simulink model "ss1_inter"  (R2019a)
settings: Solver=ode14x  StartTime=beginTime  StopTime=0.456  FixedStep=1e-4  RelTol=1e-3  EnableMultiTasking=on
model workspace (MAT data in the model file):
  Ankle_L_D = 1.86999822456
  Ankle_L_S = 0.0237763920936
  Ankle_R_D = 0.0588397140494
  Ankle_R_S = 0.739584271752
  F_C = 0.0618
  F_H = 0.107
  F_I = 0.0129
  F_L = 0.2471
  F_M = 1.2499
  F_W = 0.11
  GRF_HD = 42097.5090581
  GRF_HS = 111995.804745
  GRF_VD = 23523.4518935
  GRF_VS = 88551.3661398
  HAT_I = 4.3688
  HAT_L = 0.549
  HAT_M = 58.9182
  HAT_a = 0.2
  HAT_b = 0.13
  Hip_L_D = 0.00120944164738
  Hip_L_S = 1.91959156409
  Hip_R_D = 0.00174333284727
  Hip_R_S = 0.483982271561
  Knee_L_D = 0.900041230997
  Knee_L_S = 0.0187606009115
  Knee_R_D = 0.0722123401531
  Knee_R_S = 0.0187606009115
  M : struct (value not decoded)
  S_I = 0.073
  S_L = 0.447
  S_M = 4.0083
  S_R1 = 0.06
  S_R2 = 0.08
  T_I = 0.2042
  T_L = 0.476
  T_M = 8.62
  T_R1 = 0.08
  T_R2 = 0.1
  beginTime = 0.0166
  bodymass = 86.2
  lagStanceAnkle = [0 0 0 0 0 0]
  lagSwingAnkle = [0 0 0 0 0 0]
  lagSwingHip = [0 0 0 0 0 0]
  lagSwingKnee = [0 0 0 0 0 0]
  p_stance_ankle_i = 3.55817508048
  p_stance_hip_i = 23.7121133444
  p_stance_knee_i = -14.6552485707
  p_swing_ankle_i = -35.5709727014
  p_swing_hip_i = -19.0699177299
  p_swing_knee_i = -0.711619105868
  polyfit_stance_ankle = [23675.5212354 -31931.2429023 15252.5151968 -3621.5696911 268.973048302 -0.00762323811385]
  polyfit_swing_ankle = [-7183170.28304 10168157.4246 -5826762.40795 1748786.50975 -298844.069674 29567.8455925 -1567.7731554 24.418061318 1.56689555274]
  polyfit_swing_hip = [-184063768.654 261180473.575 -149801561.895 44513131.158 -7279965.6736 635960.536344 -25237.4588361 73.5247488612 22.0195049052]
  polyfit_swing_knee = [-121821446.299 173842986.405 -100273096.775 30000313.7158 -4970023.76394 451012.243214 -20836.4993451 353.694972881 6.37011560058]
  w_stance_ankle_i = 20.2190235478
  w_stance_hip_i = -62.2867196647
  w_stance_knee_i = -17.283984408
  w_swing_ankle_i = -338.75780931
  w_swing_hip_i = -1.73082510839
  w_swing_knee_i = 5.84839810815
  x_planar_p_i = -1.2363122322e-07
  x_planar_v_i = -5.51222083642e-05
  y_planar_p_i = -5.63070475942e-05
  y_planar_v_i = -0.0311861663822
  z_planar_p_i = 0.00649080902233
  z_planar_v_i = 3.33643661494
symbols that are objects in the model workspace (value not decoded): M
undefined symbols (not defined in the file or in its folder): X, Y, Z
libraries: nesl_utility x60, sm_lib x46, fl_lib x24, fl_ps_legacy_lib x14
(part 5 of 7)

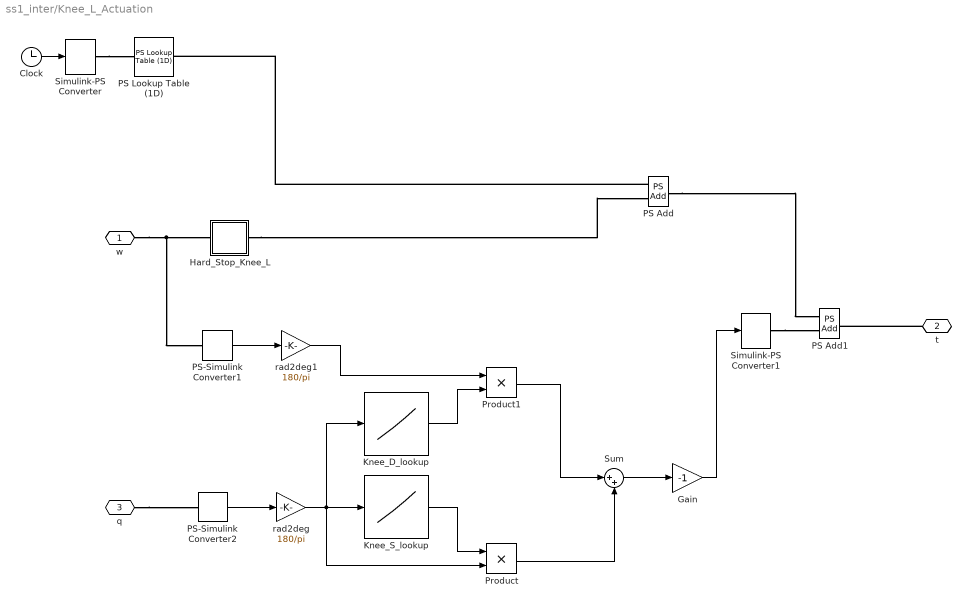
== system ss1_inter/Knee_L_Actuation ==
  Clock : Clock
  Gain : Gain  Gain=-1
  Hard_Stop_Knee_L : Subsystem  mask{upper_bound=(-p_stance_knee_i*pi)/180, lower_bound=((-140-p_stance_knee_i)*pi)/180, contact_stiffness=1e8, contact_damping=5000, initial_angular_position=0}
      mask prompts: upper_bound "Upper Bound"; lower_bound "Lower Bound"; contact_stiffness "Contact Stiffness"; contact_damping "Contact Damping"; initial_angular_position "Initial Angular Position"
  Knee_D_lookup : Lookup_n-D  NumberOfTableDimensions=1  BreakpointsForDimension1=[-140:.01:0]  Table=[exp(linspace(log(1000),log(.01),1000)), zeros(1,12000),exp(linspace(log(.01),log(1000),1001))]  RndMeth=Simplest  InputSameDT=on
  Knee_S_lookup : Lookup_n-D  NumberOfTableDimensions=1  BreakpointsForDimension1=[-140:.01:0]  Table=[exp(linspace(log(10000),log(.01),1000)), zeros(1,12000),exp(linspace(log(.01),log(10000),1001))]  RndMeth=Simplest  InputSameDT=on
  PS Add : fl_ps_legacy_lib/Legacy Physical Signals/Functions/PS Add
      settings: SourceProductName=Simscape  SourceProductBaseCode=SS
  PS Add1 : fl_ps_legacy_lib/Legacy Physical Signals/Functions/PS Add
      settings: SourceProductName=Simscape  SourceProductBaseCode=SS
  PS Lookup Table (1D) : fl_ps_legacy_lib/Legacy Physical Signals/Lookup Tables/PS Lookup Table (1D)  x=linspace(0,.3917,47)'  f=(-M.stance_knee_av/1000)*bodymass  interp_method=2  extrap_method=1
      settings: SourceProductName=Simscape  SourceProductBaseCode=SS
  PS-Simulink Converter1 : nesl_utility/PS-Simulink Converter  PhysicalDomain=network_engine_domain  SubClassName=ps_output  LeftPortType=input  RightPortType=output  PseudoPeriodic=off  Frequencies=[]  Unit=1  AffineConversion=off
  PS-Simulink Converter2 : nesl_utility/PS-Simulink Converter  PhysicalDomain=network_engine_domain  SubClassName=ps_output  LeftPortType=input  RightPortType=output  PseudoPeriodic=off  Frequencies=[]  Unit=1  AffineConversion=off
  Product : Product  RndMeth=Zero
  Product1 : Product  RndMeth=Zero
  Simulink-PS Converter : nesl_utility/Simulink-PS Converter  PhysicalDomain=network_engine_domain  SubClassName=ps_input  LeftPortType=input  RightPortType=output  PseudoPeriodic=off  Frequencies=[]  NoiseDistribution=none  NoiseParameters=[]  Unit=1  AffineConversion=off  FilteringAndDerivatives=zero  SimscapeFilterOrder=1  InputFilterTimeConstant=.001  UdotUserProvided=[]
  Simulink-PS Converter1 : nesl_utility/Simulink-PS Converter  PhysicalDomain=network_engine_domain  SubClassName=ps_input  LeftPortType=input  RightPortType=output  PseudoPeriodic=off  Frequencies=[]  NoiseDistribution=none  NoiseParameters=[]  Unit=1  AffineConversion=off  FilteringAndDerivatives=zero  SimscapeFilterOrder=1  InputFilterTimeConstant=.001  UdotUserProvided=[]
  Sum : Sum  Inputs=|++
  rad2deg : Gain  Gain=180/pi
  "rad2deg1 " : Gain  Gain=180/pi
  w : PMIOPort  Side=Right
  t : PMIOPort  Port=2  Side=Left
  q : PMIOPort  Port=3  Side=Right
  wires:
  Clock/1 -> Simulink-PS Converter/1
  PS-Simulink Converter1/1 -> "rad2deg1 "/1
  PS-Simulink Converter2/1 -> rad2deg/1
  rad2deg/1 -> Knee_S_lookup/1, Knee_D_lookup/1, Product/2
  Knee_S_lookup/1 -> Product/1
  "rad2deg1 "/1 -> Product1/1
  Product1/1 -> Sum/1
  Product/1 -> Sum/2
  Sum/1 -> Gain/1
  Gain/1 -> Simulink-PS Converter1/1
  Knee_D_lookup/1 -> Product1/2
  connections:
  Hard_Stop_Knee_L/RConn1 -- PS Add/LConn2
  w/RConn1 -- PS-Simulink Converter1/LConn1 -- Hard_Stop_Knee_L/LConn1
  Simulink-PS Converter/RConn1 -- PS Lookup Table (1D)/LConn1
  t/RConn1 -- PS Add1/RConn1
  q/RConn1 -- PS-Simulink Converter2/LConn1
  PS Add/RConn1 -- PS Add1/LConn1
  Simulink-PS Converter1/RConn1 -- PS Add1/LConn2
  PS Add/LConn1 -- PS Lookup Table (1D)/RConn1

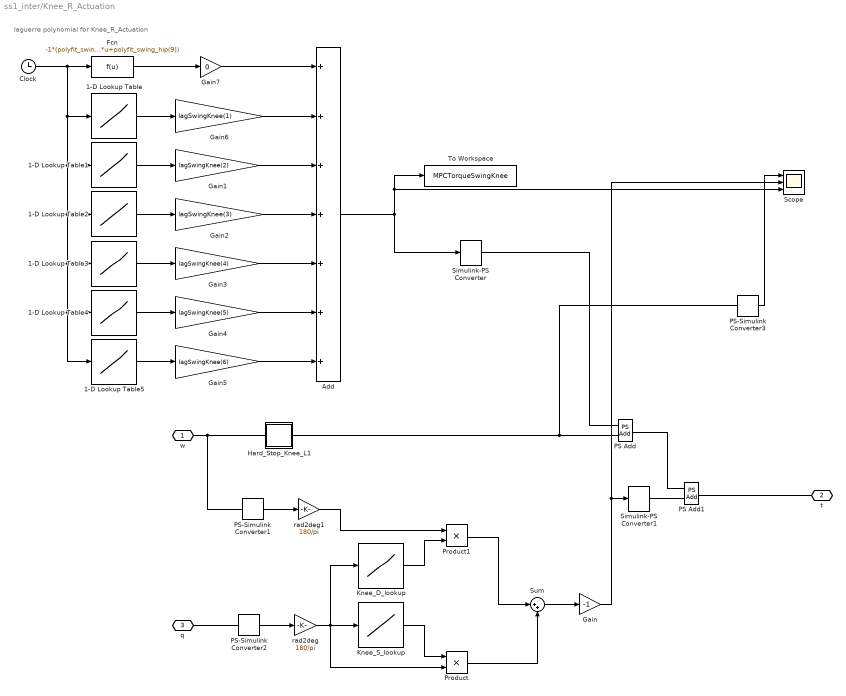
== system ss1_inter/Knee_R_Actuation ==
  note: laguerre polynomial for Knee_R_Actuation
  1-D Lookup Table : Lookup_n-D  NumberOfTableDimensions=1  BreakpointsForDimension1=|  Table=|  InternalRulePriority=Speed  RndMeth=Simplest  InputSameDT=on
      BreakpointsForDimension1=|
      | [0
      | 0.00500000000000000
      | 0.0100000000000000
      | 0.0150000000000000
      | 0.0200000000000000
      | 0.0250000000000000
      | 0.0300000000000000
      | 0.0350000000000000
      | 0.0400000000000000
      | 0.0450000000000000
      | 0.0500000000000000
      | 0.0550000000000000
      | 0.0600000000000000
      | 0.0650000000000000
      | 0.0700000000000000
      | 0.0750000000000000
      | 0.0800000000000000
      | 0.0850000000000000
      | 0.0900000000000000
      | 0.0950000000000000
      | 0.100000000000000
      | 0.105000000000000
      | 0.110000000000000
      | 0.115000000000000
      | 0.120000000000000
      | 0.125000000000000
      | 0.130000000000000
      | 0.135000000000000
      | 0.140000000000000
      | 0.145000000000000
      | 0.150000000000000
      | 0.155000000000000
      | 0.160000000000000
      | 0.165000000000000
      | 0.170000000000000
      | 0.175000000000000
      | 0.180000000000000
      | 0.185000000000000
      | 0.190000000000000
      | 0.195000000000000
      | 0.200000000000000
      | 0.205000000000000
      | 0.210000000000000
      | 0.215000000000000
      | 0.220000000000000
      | 0.225000000000000
      | 0.230000000000000
      | 0.235000000000000
      | 0.240000000000000
      | 0.245000000000000
      | 0.250000000000000
      | 0.255000000000000
      | 0.260000000000000
      | 0.265000000000000
      | 0.270000000000000
      | 0.275000000000000
      | 0.280000000000000
      | 0.285000000000000
      | 0.290000000000000
      | 0.295000000000000
      | 0.300000000000000
      | 0.305000000000000
      | 0.310000000000000
      | 0.315000000000000
      | 0.320000000000000
      | 0.325000000000000
      | 0.330000000000000
      | 0.335000000000000
      | 0.340000000000000
      | 0.345000000000000
      | 0.350000000000000
      | 0.355000000000000
      | 0.360000000000000
      | 0.365000000000000
      | 0.370000000000000
      | 0.375000000000000
      | 0.380000000000000
      | 0.385000000000000
      | 0.390000000000000
      | 0.395000000000000
      | 0.400000000000000
      | 0.405000000000000
      | 0.410000000000000
      | 0.415000000000000
      | 0.420000000000000
      | 0.425000000000000
      | 0.430000000000000
      | 0.435000000000000
      | 0.440000000000000
      | 0.445000000000000
      | 0.450000000000000
      | 0.455000000000000
      | 0.460000000000000
      | 0.465000000000000
      | 0.470000000000000
      | 0.475000000000000
      | 0.480000000000000
      | 0.485000000000000
      | 0.490000000000000
      | 0.495000000000000
      | 0.500000000000000]
      Table=|
      | [1
      | 0.800000000000000
      | 0.640000000000000
      | 0.512000000000000
      | 0.409600000000000
      | 0.327680000000000
      | 0.262144000000000
      | 0.209715200000000
      | 0.167772160000000
      | 0.134217728000000
      | 0.107374182400000
      | 0.0858993459200001
      | 0.0687194767360000
      | 0.0549755813888000
      | 0.0439804651110400
      | 0.0351843720888320
      | 0.0281474976710656
      | 0.0225179981368525
      | 0.0180143985094820
      | 0.0144115188075856
      | 0.0115292150460685
      | 0.00922337203685479
      | 0.00737869762948383
      | 0.00590295810358706
      | 0.00472236648286965
      | 0.00377789318629572
      | 0.00302231454903658
      | 0.00241785163922926
      | 0.00193428131138341
      | 0.00154742504910673
      | 0.00123794003928538
      | 0.000990352031428306
      | 0.000792281625142645
      | 0.000633825300114116
      | 0.000507060240091293
      | 0.000405648192073034
      | 0.000324518553658427
      | 0.000259614842926742
      | 0.000207691874341394
      | 0.000166153499473115
      | 0.000132922799578492
      | 0.000106338239662794
      | 8.50705917302348e-05
      | 6.80564733841879e-05
      | 5.44451787073503e-05
      | 4.35561429658802e-05
      | 3.48449143727042e-05
      | 2.78759314981633e-05
      | 2.23007451985307e-05
      | 1.78405961588245e-05
      | 1.42724769270596e-05
      | 1.14179815416477e-05
      | 9.13438523331817e-06
      | 7.30750818665453e-06
      | 5.84600654932363e-06
      | 4.67680523945890e-06
      | 3.74144419156712e-06
      | 2.99315535325370e-06
      | 2.39452428260296e-06
      | 1.91561942608237e-06
      | 1.53249554086589e-06
      | 1.22599643269272e-06
      | 9.80797146154172e-07
      | 7.84637716923338e-07
      | 6.27710173538670e-07
      | 5.02168138830936e-07
      | 4.01734511064749e-07
      | 3.21387608851799e-07
      | 2.57110087081439e-07
      | 2.05688069665152e-07
      | 1.64550455732121e-07
      | 1.31640364585697e-07
      | 1.05312291668558e-07
      | 8.42498333348461e-08
      | 6.73998666678769e-08
      | 5.39198933343015e-08
      | 4.31359146674412e-08
      | 3.45087317339530e-08
      | 2.76069853871624e-08
      | 2.20855883097299e-08
      | 1.76684706477839e-08
      | 1.41347765182271e-08
      | 1.13078212145817e-08
      | 9.04625697166537e-09
      | 7.23700557733230e-09
      | 5.78960446186584e-09
      | 4.63168356949267e-09
      | 3.70534685559414e-09
      | 2.96427748447531e-09
      | 2.37142198758025e-09
      | 1.89713759006420e-09
      | 1.51771007205136e-09
      | 1.21416805764109e-09
      | 9.71334446112870e-10
      | 7.77067556890296e-10
      | 6.21654045512237e-10
      | 4.97323236409790e-10
      | 3.97858589127832e-10
      | 3.18286871302265e-10
      | 2.54629497041812e-10
      | 2.03703597633450e-10]
  1-D Lookup Table1 : Lookup_n-D  NumberOfTableDimensions=1  BreakpointsForDimension1=|  Table=|  InternalRulePriority=Speed  RndMeth=Simplest  InputSameDT=on
      BreakpointsForDimension1=|
      | [0
      | 0.00500000000000000
      | 0.0100000000000000
      | 0.0150000000000000
      | 0.0200000000000000
      | 0.0250000000000000
      | 0.0300000000000000
      | 0.0350000000000000
      | 0.0400000000000000
      | 0.0450000000000000
      | 0.0500000000000000
      | 0.0550000000000000
      | 0.0600000000000000
      | 0.0650000000000000
      | 0.0700000000000000
      | 0.0750000000000000
      | 0.0800000000000000
      | 0.0850000000000000
      | 0.0900000000000000
      | 0.0950000000000000
      | 0.100000000000000
      | 0.105000000000000
      | 0.110000000000000
      | 0.115000000000000
      | 0.120000000000000
      | 0.125000000000000
      | 0.130000000000000
      | 0.135000000000000
      | 0.140000000000000
      | 0.145000000000000
      | 0.150000000000000
      | 0.155000000000000
      | 0.160000000000000
      | 0.165000000000000
      | 0.170000000000000
      | 0.175000000000000
      | 0.180000000000000
      | 0.185000000000000
      | 0.190000000000000
      | 0.195000000000000
      | 0.200000000000000
      | 0.205000000000000
      | 0.210000000000000
      | 0.215000000000000
      | 0.220000000000000
      | 0.225000000000000
      | 0.230000000000000
      | 0.235000000000000
      | 0.240000000000000
      | 0.245000000000000
      | 0.250000000000000
      | 0.255000000000000
      | 0.260000000000000
      | 0.265000000000000
      | 0.270000000000000
      | 0.275000000000000
      | 0.280000000000000
      | 0.285000000000000
      | 0.290000000000000
      | 0.295000000000000
      | 0.300000000000000
      | 0.305000000000000
      | 0.310000000000000
      | 0.315000000000000
      | 0.320000000000000
      | 0.325000000000000
      | 0.330000000000000
      | 0.335000000000000
      | 0.340000000000000
      | 0.345000000000000
      | 0.350000000000000
      | 0.355000000000000
      | 0.360000000000000
      | 0.365000000000000
      | 0.370000000000000
      | 0.375000000000000
      | 0.380000000000000
      | 0.385000000000000
      | 0.390000000000000
      | 0.395000000000000
      | 0.400000000000000
      | 0.405000000000000
      | 0.410000000000000
      | 0.415000000000000
      | 0.420000000000000
      | 0.425000000000000
      | 0.430000000000000
      | 0.435000000000000
      | 0.440000000000000
      | 0.445000000000000
      | 0.450000000000000
      | 0.455000000000000
      | 0.460000000000000
      | 0.465000000000000
      | 0.470000000000000
      | 0.475000000000000
      | 0.480000000000000
      | 0.485000000000000
      | 0.490000000000000
      | 0.495000000000000
      | 0.500000000000000]
      Table=|
      | [-0.800000000000000
      | -0.280000000000000
      | 0.0639999999999997
      | 0.281600000000000
      | 0.409600000000000
      | 0.475136000000000
      | 0.498073600000000
      | 0.492830720000000
      | 0.469762048000000
      | 0.436207616000000
      | 0.397284474880000
      | 0.356482285568000
      | 0.316109592985600
      | 0.277626686013440
      | 0.241892558110720
      | 0.209347013928550
      | 0.180143985094820
      | 0.154248287237440
      | 0.131505109119219
      | 0.111689270758788
      | 0.0945395633777615
      | 0.0797821681187939
      | 0.0671461484283028
      | 0.0563732498892564
      | 0.0472236648286965
      | 0.0394789837967903
      | 0.0329432285844987
      | 0.0274426161052521
      | 0.0228245194743242
      | 0.0189559568515574
      | 0.0157218384989243
      | 0.0130231292132822
      | 0.0107750301019400
      | 0.00890524546660332
      | 0.00735237348132374
      | 0.00606444047149186
      | 0.00499758572633978
      | 0.00411489526038886
      | 0.00338537755176471
      | 0.00278307111617467
      | 0.00228627215275006
      | 0.00187686993004830
      | 0.00153977771031725
      | 0.00126244758127668
      | 0.00103445839543965
      | 0.000847166980686370
      | 0.000693413796016813
      | 0.000567275205987624
      | 0.000463855500129438
      | 0.000379112668375021
      | 0.000309712749317194
      | 0.000252908291147497
      | 0.000206437106272991
      | 0.000168438063702387
      | 0.000137381153909105
      | 0.000112009485485041
      | 9.12912382742378e-05
      | 7.43799105283544e-05
      | 6.05814643498548e-05
      | 4.93272002216209e-05
      | 4.01513831706864e-05
      | 3.26728049312609e-05
      | 2.65796026607781e-05
      | 2.16167691012380e-05
      | 1.75758848590828e-05
      | 1.42866835497401e-05
      | 1.16101273697712e-05
      | 9.43272631980031e-06
      | 7.66188059502689e-06
      | 6.22206410737083e-06
      | 5.05169899097612e-06
      | 4.10059735684446e-06
      | 3.32786841672642e-06
      | 2.70020715838182e-06
      | 2.19049566670600e-06
      | 1.77666048536523e-06
      | 1.44073954989254e-06
      | 1.16812056919431e-06
      | 9.46919598779670e-07
      | 7.67474193763114e-07
      | 6.21930166801994e-07
      | 5.03904782874798e-07
      | 4.08212345846400e-07
      | 3.30640692314369e-07
      | 2.67769206361295e-07
      | 2.16820687096876e-07
      | 1.75540807283772e-07
      | 1.42100051912035e-07
      | 1.15013966397642e-07
      | 9.30783130125247e-08
      | 7.53163623255487e-08
      | 6.09360593928621e-08
      | 4.92952231402281e-08
      | 3.98732790129333e-08
      | 3.22483036109473e-08
      | 2.60783872092383e-08
      | 2.10865052237751e-08
      | 1.70482405441276e-08
      | 1.37818215273881e-08
      | 1.11400404955793e-08
      | 9.00369901539848e-09]
  1-D Lookup Table2 : Lookup_n-D  NumberOfTableDimensions=1  BreakpointsForDimension1=|  Table=|  InternalRulePriority=Speed  RndMeth=Simplest  InputSameDT=on
      BreakpointsForDimension1=|
      | [0
      | 0.00500000000000000
      | 0.0100000000000000
      | 0.0150000000000000
      | 0.0200000000000000
      | 0.0250000000000000
      | 0.0300000000000000
      | 0.0350000000000000
      | 0.0400000000000000
      | 0.0450000000000000
      | 0.0500000000000000
      | 0.0550000000000000
      | 0.0600000000000000
      | 0.0650000000000000
      | 0.0700000000000000
      | 0.0750000000000000
      | 0.0800000000000000
      | 0.0850000000000000
      | 0.0900000000000000
      | 0.0950000000000000
      | 0.100000000000000
      | 0.105000000000000
      | 0.110000000000000
      | 0.115000000000000
      | 0.120000000000000
      | 0.125000000000000
      | 0.130000000000000
      | 0.135000000000000
      | 0.140000000000000
      | 0.145000000000000
      | 0.150000000000000
      | 0.155000000000000
      | 0.160000000000000
      | 0.165000000000000
      | 0.170000000000000
      | 0.175000000000000
      | 0.180000000000000
      | 0.185000000000000
      | 0.190000000000000
      | 0.195000000000000
      | 0.200000000000000
      | 0.205000000000000
      | 0.210000000000000
      | 0.215000000000000
      | 0.220000000000000
      | 0.225000000000000
      | 0.230000000000000
      | 0.235000000000000
      | 0.240000000000000
      | 0.245000000000000
      | 0.250000000000000
      | 0.255000000000000
      | 0.260000000000000
      | 0.265000000000000
      | 0.270000000000000
      | 0.275000000000000
      | 0.280000000000000
      | 0.285000000000000
      | 0.290000000000000
      | 0.295000000000000
      | 0.300000000000000
      | 0.305000000000000
      | 0.310000000000000
      | 0.315000000000000
      | 0.320000000000000
      | 0.325000000000000
      | 0.330000000000000
      | 0.335000000000000
      | 0.340000000000000
      | 0.345000000000000
      | 0.350000000000000
      | 0.355000000000000
      | 0.360000000000000
      | 0.365000000000000
      | 0.370000000000000
      | 0.375000000000000
      | 0.380000000000000
      | 0.385000000000000
      | 0.390000000000000
      | 0.395000000000000
      | 0.400000000000000
      | 0.405000000000000
      | 0.410000000000000
      | 0.415000000000000
      | 0.420000000000000
      | 0.425000000000000
      | 0.430000000000000
      | 0.435000000000000
      | 0.440000000000000
      | 0.445000000000000
      | 0.450000000000000
      | 0.455000000000000
      | 0.460000000000000
      | 0.465000000000000
      | 0.470000000000000
      | 0.475000000000000
      | 0.480000000000000
      | 0.485000000000000
      | 0.490000000000000
      | 0.495000000000000
      | 0.500000000000000]
      Table=|
      | [0.640000000000000
      | -0.0639999999999997
      | -0.382400000000000
      | -0.467200000000000
      | -0.419840000000000
      | -0.306380800000000
      | -0.168427520000000
      | -0.0309329920000004
      | 0.0922746879999996
      | 0.194615705600000
      | 0.274072600576000
      | 0.331356726886400
      | 0.368679992688640
      | 0.388952238325760
      | 0.395274430185472
      | 0.390634491116257
      | 0.377739418745700
      | 0.358936890301428
      | 0.336193712183208
      | 0.311108662258754
      | 0.284944549863582
      | 0.258669468773592
      | 0.233000824395025
      | 0.208448208032918
      | 0.185352884452634
      | 0.163922785353371
      | 0.144262629211888
      | 0.126399239069808
      | 0.110302391781639
      | 0.0959016674183893
      | 0.0830998199871294
      | 0.0717831911180021
      | 0.0618296580261319
      | 0.0531145601495628
      | 0.0455149948011946
      | 0.0389128169450859
      | 0.0331966254464888
      | 0.0282629698752197
      | 0.0240169691191529
      | 0.0203724959541473
      | 0.0172520501572924
      | 0.0145864163345454
      | 0.0123141808294308
      | 0.0103811643088405
      | 0.00873981231199740
      | 0.00734857466048848
      | 0.00617129567226370
      | 0.00517663016903767
      | 0.00433749494111421
      | 0.00363056131832079
      | 0.00303579152357790
      | 0.00253601933526152
      | 0.00211657407433832
      | 0.00176494591478174
      | 0.00147048987240049
      | 0.00122416546344147
      | 0.00101830886561882
      | 0.000846434402346613
      | 0.000703062260925761
      | 0.000583569512913167
      | 0.000484061704015605
      | 0.000401262502438162
      | 0.000332419124753168
      | 0.000275221487182322
      | 0.000227733250959829
      | 0.000188333138787154
      | 0.000155665092683647
      | 0.000128596020460848
      | 0.000106180038212457
      | 8.76282598790961e-05
      | 7.22833128178668e-05
      | 5.95978713597940e-05
      | 4.91165997112986e-05
      | 4.04609824590598e-05
      | 3.33165965922649e-05
      | 2.74224445522257e-05
      | 2.25620244872318e-05
      | 1.85558626843225e-05
      | 1.52552750376286e-05
      | 1.25371602738720e-05
      | 1.02996582794192e-05
      | 8.45853296403748e-06
      | 6.94416127742766e-06
      | 5.69902881393703e-06
      | 4.67564837837496e-06
      | 3.83483135938376e-06
      | 3.14425312877687e-06
      | 2.57726326877564e-06
      | 2.11189949381443e-06
      | 1.73007091103917e-06
      | 1.41688195198342e-06
      | 1.16007307639800e-06
      | 9.49558341999076e-07
      | 7.77043273529142e-07
      | 6.35709254947489e-07
      | 5.19952997801548e-07
      | 4.25171581271457e-07
      | 3.47585177805638e-07
      | 2.84090925566728e-07
      | 2.32142529584307e-07
      | 1.89651104950706e-07]
  1-D Lookup Table3 : Lookup_n-D  NumberOfTableDimensions=1  BreakpointsForDimension1=|  Table=|  InternalRulePriority=Speed  RndMeth=Simplest  InputSameDT=on
      BreakpointsForDimension1=|
      | [0
      | 0.00500000000000000
      | 0.0100000000000000
      | 0.0150000000000000
      | 0.0200000000000000
      | 0.0250000000000000
      | 0.0300000000000000
      | 0.0350000000000000
      | 0.0400000000000000
      | 0.0450000000000000
      | 0.0500000000000000
      | 0.0550000000000000
      | 0.0600000000000000
      | 0.0650000000000000
      | 0.0700000000000000
      | 0.0750000000000000
      | 0.0800000000000000
      | 0.0850000000000000
      | 0.0900000000000000
      | 0.0950000000000000
      | 0.100000000000000
      | 0.105000000000000
      | 0.110000000000000
      | 0.115000000000000
      | 0.120000000000000
      | 0.125000000000000
      | 0.130000000000000
      | 0.135000000000000
      | 0.140000000000000
      | 0.145000000000000
      | 0.150000000000000
      | 0.155000000000000
      | 0.160000000000000
      | 0.165000000000000
      | 0.170000000000000
      | 0.175000000000000
      | 0.180000000000000
      | 0.185000000000000
      | 0.190000000000000
      | 0.195000000000000
      | 0.200000000000000
      | 0.205000000000000
      | 0.210000000000000
      | 0.215000000000000
      | 0.220000000000000
      | 0.225000000000000
      | 0.230000000000000
      | 0.235000000000000
      | 0.240000000000000
      | 0.245000000000000
      | 0.250000000000000
      | 0.255000000000000
      | 0.260000000000000
      | 0.265000000000000
      | 0.270000000000000
      | 0.275000000000000
      | 0.280000000000000
      | 0.285000000000000
      | 0.290000000000000
      | 0.295000000000000
      | 0.300000000000000
      | 0.305000000000000
      | 0.310000000000000
      | 0.315000000000000
      | 0.320000000000000
      | 0.325000000000000
      | 0.330000000000000
      | 0.335000000000000
      | 0.340000000000000
      | 0.345000000000000
      | 0.350000000000000
      | 0.355000000000000
      | 0.360000000000000
      | 0.365000000000000
      | 0.370000000000000
      | 0.375000000000000
      | 0.380000000000000
      | 0.385000000000000
      | 0.390000000000000
      | 0.395000000000000
      | 0.400000000000000
      | 0.405000000000000
      | 0.410000000000000
      | 0.415000000000000
      | 0.420000000000000
      | 0.425000000000000
      | 0.430000000000000
      | 0.435000000000000
      | 0.440000000000000
      | 0.445000000000000
      | 0.450000000000000
      | 0.455000000000000
      | 0.460000000000000
      | 0.465000000000000
      | 0.470000000000000
      | 0.475000000000000
      | 0.480000000000000
      | 0.485000000000000
      | 0.490000000000000
      | 0.495000000000000
      | 0.500000000000000]
      Table=|
      | [-0.512000000000000
      | 0.281600000000000
      | 0.467200000000000
      | 0.365120000000000
      | 0.160768000000000
      | -0.0461209599999997
      | -0.208535552000000
      | -0.310509568000000
      | -0.353160396800000
      | -0.345946193920000
      | -0.301399329996800
      | -0.232132244930560
      | -0.149293063208960
      | -0.0619162485391363
      | 0.0231996953460732
      | 0.101326593569325
      | 0.169504230975157
      | 0.226193291284683
      | 0.270936553582609
      | 0.304056025242291
      | 0.326397842561721
      | 0.339127248894085
      | 0.343570608372840
      | 0.341098744666963
      | 0.333044896204382
      | 0.320650573133442
      | 0.305033140490614
      | 0.287169750348533
      | 0.267893125923323
      | 0.247895558585586
      | 0.227738258297155
      | 0.207863873730451
      | 0.188610563681458
      | 0.170226460851648
      | 0.152883732989925
      | 0.136691727637066
      | 0.121708898697548
      | 0.107953368504351
      | 0.0954120893833785
      | 0.0840486438625378
      | 0.0738097709183436
      | 0.0646307338243310
      | 0.0564396587304655
      | 0.0491609763667308
      | 0.0427180955526273
      | 0.0370354290257084
      | 0.0320398813432443
      | 0.0276618966116290
      | 0.0238361515054495
      | 0.0205019670908172
      | 0.0176035017721122
      | 0.0150897774730585
      | 0.0129145820542376
      | 0.0110362829859030
      | 0.00941758040558377
      | 0.00802522182611433
      | 0.00682969583183787
      | 0.00580491800921183
      | 0.00492791900097547
      | 0.00417854185137560
      | 0.00353915363080116
      | 0.00299437460670601
      | 0.00253082688800043
      | 0.00213690344540766
      | 0.00180255764274058
      | 0.00151911285412257
      | 0.00127909134793830
      | 0.00107606135466560
      | 0.000904501073623366
      | 0.000759678289207873
      | 0.000637544240991101
      | 0.000534640408522913
      | 0.000448016918409085
      | 0.000375161348471319
      | 0.000313936783962303
      | 0.000262528068120327
      | 0.000219395279458702
      | 0.000183233557906735
      | 0.000152938488979608
      | 0.000127576338002217
      | 0.000106358504052111
      | 8.86196351498776e-05
      | 7.37989120619974e-05
      | 6.14240678758760e-05
      | 5.10977644119378e-05
      | 4.24859948204182e-05
      | 3.53082247126969e-05
      | 2.93290222839138e-05
      | 2.43509615008552e-05
      | 2.02086119656672e-05
      | 1.67634549219862e-05
      | 1.38995874284540e-05
      | 1.15200963455619e-05
      | 9.54400079962531e-06
      | 7.90367650927140e-06
      | 6.54268806412337e-06
      | 5.41396618408308e-06
      | 4.47827638629341e-06
      | 3.70293354638698e-06
      | 3.06072373900887e-06
      | 2.52900063683084e-06]
  1-D Lookup Table4 : Lookup_n-D  NumberOfTableDimensions=1  BreakpointsForDimension1=|  Table=|  InternalRulePriority=Speed  RndMeth=Simplest  InputSameDT=on
      BreakpointsForDimension1=|
      | [0
      | 0.00500000000000000
      | 0.0100000000000000
      | 0.0150000000000000
      | 0.0200000000000000
      | 0.0250000000000000
      | 0.0300000000000000
      | 0.0350000000000000
      | 0.0400000000000000
      | 0.0450000000000000
      | 0.0500000000000000
      | 0.0550000000000000
      | 0.0600000000000000
      | 0.0650000000000000
      | 0.0700000000000000
      | 0.0750000000000000
      | 0.0800000000000000
      | 0.0850000000000000
      | 0.0900000000000000
      | 0.0950000000000000
      | 0.100000000000000
      | 0.105000000000000
      | 0.110000000000000
      | 0.115000000000000
      | 0.120000000000000
      | 0.125000000000000
      | 0.130000000000000
      | 0.135000000000000
      | 0.140000000000000
      | 0.145000000000000
      | 0.150000000000000
      | 0.155000000000000
      | 0.160000000000000
      | 0.165000000000000
      | 0.170000000000000
      | 0.175000000000000
      | 0.180000000000000
      | 0.185000000000000
      | 0.190000000000000
      | 0.195000000000000
      | 0.200000000000000
      | 0.205000000000000
      | 0.210000000000000
      | 0.215000000000000
      | 0.220000000000000
      | 0.225000000000000
      | 0.230000000000000
      | 0.235000000000000
      | 0.240000000000000
      | 0.245000000000000
      | 0.250000000000000
      | 0.255000000000000
      | 0.260000000000000
      | 0.265000000000000
      | 0.270000000000000
      | 0.275000000000000
      | 0.280000000000000
      | 0.285000000000000
      | 0.290000000000000
      | 0.295000000000000
      | 0.300000000000000
      | 0.305000000000000
      | 0.310000000000000
      | 0.315000000000000
      | 0.320000000000000
      | 0.325000000000000
      | 0.330000000000000
      | 0.335000000000000
      | 0.340000000000000
      | 0.345000000000000
      | 0.350000000000000
      | 0.355000000000000
      | 0.360000000000000
      | 0.365000000000000
      | 0.370000000000000
      | 0.375000000000000
      | 0.380000000000000
      | 0.385000000000000
      | 0.390000000000000
      | 0.395000000000000
      | 0.400000000000000
      | 0.405000000000000
      | 0.410000000000000
      | 0.415000000000000
      | 0.420000000000000
      | 0.425000000000000
      | 0.430000000000000
      | 0.435000000000000
      | 0.440000000000000
      | 0.445000000000000
      | 0.450000000000000
      | 0.455000000000000
      | 0.460000000000000
      | 0.465000000000000
      | 0.470000000000000
      | 0.475000000000000
      | 0.480000000000000
      | 0.485000000000000
      | 0.490000000000000
      | 0.495000000000000
      | 0.500000000000000]
      Table=|
      | [0.409600000000000
      | -0.409600000000000
      | -0.419840000000000
      | -0.160768000000000
      | 0.107891200000000
      | 0.283977728000000
      | 0.347889664000000
      | 0.318183833600000
      | 0.226565816320000
      | 0.104849211392000
      | -0.0209473608089596
      | -0.132451422699520
      | -0.218658932523008
      | -0.274687210396057
      | -0.300225773132841
      | -0.298042198015659
      | -0.272710549623328
      | -0.229618841751252
      | -0.174251024982406
      | -0.111709086597149
      | -0.0464295180848049
      | 0.0179524289786089
      | 0.0786327053787003
      | 0.133597776942230
      | 0.181541049257242
      | 0.221757277103421
      | 0.254029882423688
      | 0.278521246150738
      | 0.295672246530465
      | 0.306114476279226
      | 0.310596532971243
      | 0.309924385689788
      | 0.304914931337116
      | 0.296361340069832
      | 0.285008546515573
      | 0.271537188092731
      | 0.256554359153213
      | 0.240589691216637
      | 0.224095449970958
      | 0.207449534270115
      | 0.190960454543955
      | 0.174873547494043
      | 0.159377844835193
      | 0.144613153505235
      | 0.130677022728817
      | 0.117631370515114
      | 0.105508620363204
      | 0.0943172603445045
      | 0.0840467836828730
      | 0.0746720047790942
      | 0.0661567694964027
      | 0.0584570953907876
      | 0.0515237881422985
      | 0.0453045861793540
      | 0.0397458876049192
      | 0.0347941130286277
      | 0.0303967555835462
      | 0.0265031658913053
      | 0.0230651155214757
      | 0.0200371779370556
      | 0.0173769612963791
      | 0.0150452229825397
      | 0.0130058914823374
      | 0.0112260173175442
      | 0.00967567118525057
      | 0.00832780430764298
      | 0.00715808322188632
      | 0.00614470884171487
      | 0.00526822756913881
      | 0.00451134049756811
      | 0.00385871529446948
      | 0.00329680414974836
      | 0.00281367019359433
      | 0.00239882399450749
      | 0.00204307111690747
      | 0.00173837122299202
      | 0.00147770882294698
      | 0.00125497549149090
      | 0.00106486315991577
      | 0.000902767946510448
      | 0.000764703891968888
      | 0.000647225909507318
      | 0.000547361233106134
      | 0.000462548644246204
      | 0.000390584771743289
      | 0.000329576785950234
      | 0.000277900843810448
      | 0.000234165681933924
      | 0.000197180798630369
      | 0.000165928710832617
      | 0.000139540816694172
      | 0.000117276438334560
      | 9.85046610196528e-05
      | 8.26886245215839e-05
      | 6.93719592094753e-05
      | 5.81670934255530e-05
      | 4.87451898572993e-05
      | 4.08274969608878e-05
      | 3.41779271178940e-05
      | 2.85966962494951e-05
      | 2.39148802291403e-05]
  1-D Lookup Table5 : Lookup_n-D  NumberOfTableDimensions=1  BreakpointsForDimension1=|  Table=|  InternalRulePriority=Speed  RndMeth=Simplest  InputSameDT=on
      BreakpointsForDimension1=|
      | [0
      | 0.00500000000000000
      | 0.0100000000000000
      | 0.0150000000000000
      | 0.0200000000000000
      | 0.0250000000000000
      | 0.0300000000000000
      | 0.0350000000000000
      | 0.0400000000000000
      | 0.0450000000000000
      | 0.0500000000000000
      | 0.0550000000000000
      | 0.0600000000000000
      | 0.0650000000000000
      | 0.0700000000000000
      | 0.0750000000000000
      | 0.0800000000000000
      | 0.0850000000000000
      | 0.0900000000000000
      | 0.0950000000000000
      | 0.100000000000000
      | 0.105000000000000
      | 0.110000000000000
      | 0.115000000000000
      | 0.120000000000000
      | 0.125000000000000
      | 0.130000000000000
      | 0.135000000000000
      | 0.140000000000000
      | 0.145000000000000
      | 0.150000000000000
      | 0.155000000000000
      | 0.160000000000000
      | 0.165000000000000
      | 0.170000000000000
      | 0.175000000000000
      | 0.180000000000000
      | 0.185000000000000
      | 0.190000000000000
      | 0.195000000000000
      | 0.200000000000000
      | 0.205000000000000
      | 0.210000000000000
      | 0.215000000000000
      | 0.220000000000000
      | 0.225000000000000
      | 0.230000000000000
      | 0.235000000000000
      | 0.240000000000000
      | 0.245000000000000
      | 0.250000000000000
      | 0.255000000000000
      | 0.260000000000000
      | 0.265000000000000
      | 0.270000000000000
      | 0.275000000000000
      | 0.280000000000000
      | 0.285000000000000
      | 0.290000000000000
      | 0.295000000000000
      | 0.300000000000000
      | 0.305000000000000
      | 0.310000000000000
      | 0.315000000000000
      | 0.320000000000000
      | 0.325000000000000
      | 0.330000000000000
      | 0.335000000000000
      | 0.340000000000000
      | 0.345000000000000
      | 0.350000000000000
      | 0.355000000000000
      | 0.360000000000000
      | 0.365000000000000
      | 0.370000000000000
      | 0.375000000000000
      | 0.380000000000000
      | 0.385000000000000
      | 0.390000000000000
      | 0.395000000000000
      | 0.400000000000000
      | 0.405000000000000
      | 0.410000000000000
      | 0.415000000000000
      | 0.420000000000000
      | 0.425000000000000
      | 0.430000000000000
      | 0.435000000000000
      | 0.440000000000000
      | 0.445000000000000
      | 0.450000000000000
      | 0.455000000000000
      | 0.460000000000000
      | 0.465000000000000
      | 0.470000000000000
      | 0.475000000000000
      | 0.480000000000000
      | 0.485000000000000
      | 0.490000000000000
      | 0.495000000000000
      | 0.500000000000000]
      Table=|
      | [-0.327680000000000
      | 0.475136000000000
      | 0.306380800000000
      | -0.0461209599999997
      | -0.283977728000000
      | -0.346473164800000
      | -0.271512535040000
      | -0.123867430912001
      | 0.0378372358143994
      | 0.172956235857919
      | 0.259972088725504
      | 0.292991448331059
      | 0.276868881983734
      | 0.222585941380825
      | 0.143562161214875
      | 0.0530577142515869
      | -0.0374275869157272
      | -0.118957545754908
      | -0.185384058369254
      | -0.233191002400090
      | -0.261118274049377
      | -0.269686080507194
      | -0.260702599730106
      | -0.236807595959169
      | -0.201081139230898
      | -0.156729683810214
      | -0.106850375883700
      | -0.0542674152038624
      | -0.00143048323672425
      | 0.0496362789177043
      | 0.0973462730363951
      | 0.140534042848529
      | 0.178419674898919
      | 0.210561599200385
      | 0.236803782217681
      | 0.257221821815534
      | 0.272071158222588
      | 0.281739532757973
      | 0.286704957446249
      | 0.287499788511866
      | 0.284681001444443
      | 0.278806417704275
      | 0.270416405789309
      | 0.260020446662452
      | 0.248087892652143
      | 0.235042240438440
      | 0.221258266575302
      | 0.207061425347843
      | 0.192728973676480
      | 0.178492358800782
      | 0.164540476222598
      | 0.151023474161851
      | 0.138056844206429
      | 0.125725594563959
      | 0.114088351746586
      | 0.103181278579286
      | 0.0930217314252192
      | 0.0836116080106772
      | 0.0749403598826666
      | 0.0669876610779645
      | 0.0597257377623239
      | 0.0531213731202065
      | 0.0471376082928350
      | 0.0417351642625700
      | 0.0368736117793997
      | 0.0325123171626560
      | 0.0286111914602587
      | 0.0251312693167214
      | 0.0220351422397809
      | 0.0192872689629091
      | 0.0168541834323198
      | 0.0147046187205266
      | 0.0128095629712942
      | 0.0111422613750237
      | 0.00967817620100047
      | 0.00839491509931423
      | 0.00727213624408582
      | 0.00629143742502292
      | 0.00543623490357662
      | 0.00469163672556871
      | 0.00404431421339030
      | 0.00348237453507527
      | 0.00299523655108263
      | 0.00257351155857528
      | 0.00220889007371179
      | 0.00189403540195254
      | 0.00162248443246391
      | 0.00138855584423443
      | 0.00118726571841718
      | 0.00101425040469802
      | 0.000865696381235692
      | 0.000738276771015077
      | 0.000629094126330900
      | 0.000535629062467106
      | 0.000455694307127688
      | 0.000387393730171184
      | 0.000329085925676660
      | 0.000279351932829917
      | 0.000236966701530506
      | 0.000200873931342703
      | 0.000170163937140345]
  Add : Sum  Inputs=+++++++
  Clock : Clock
  Fcn : Fcn  Expr=-1*(polyfit_swing_hip(1)*u^8+polyfit_swing_hip(2)*u^7+polyfit_swing_hip(3)*u^6+polyfit_swing_hip(4)*u^5+polyfit_swing_hip(5)*u^4+polyfit_swing_hip(6)*u^3+polyfit_swing_hip(7)*u^2+polyfit_swing_hip(8)*u+polyfit_swing_hip(9))
  Gain : Gain  Gain=-1
  Gain1 : Gain  Gain=lagSwingKnee(2)
  Gain2 : Gain  Gain=lagSwingKnee(3)
  Gain3 : Gain  Gain=lagSwingKnee(4)
  Gain4 : Gain  Gain=lagSwingKnee(5)
  Gain5 : Gain  Gain=lagSwingKnee(6)
  Gain6 : Gain  Gain=lagSwingKnee(1)
  Gain7 : Gain  Gain=0
  Hard_Stop_Knee_L1 : Subsystem  mask{upper_bound=(-p_swing_knee_i*pi)/180, lower_bound=((-140-p_swing_knee_i)*pi)/180, contact_stiffness=1e8, contact_damping=5000, initial_angular_position=0}
      mask prompts: upper_bound "Upper Bound"; lower_bound "Lower Bound"; contact_stiffness "Contact Stiffness"; contact_damping "Contact Damping"; initial_angular_position "Initial Angular Position"
  Knee_D_lookup : Lookup_n-D  NumberOfTableDimensions=1  BreakpointsForDimension1=[-140:.01:0]  Table=[exp(linspace(log(1000),log(.01),1000)), zeros(1,12000),exp(linspace(log(.01),log(1000),1001))]  RndMeth=Simplest  InputSameDT=on
  Knee_S_lookup : Lookup_n-D  NumberOfTableDimensions=1  BreakpointsForDimension1=[-140:.01:0]  Table=[exp(linspace(log(10000),log(.01),1000)), zeros(1,12000),exp(linspace(log(.01),log(10000),1001))]  RndMeth=Simplest  InputSameDT=on
  PS Add : fl_ps_legacy_lib/Legacy Physical Signals/Functions/PS Add
      settings: SourceProductName=Simscape  SourceProductBaseCode=SS
  PS Add1 : fl_ps_legacy_lib/Legacy Physical Signals/Functions/PS Add
      settings: SourceProductName=Simscape  SourceProductBaseCode=SS
  PS-Simulink Converter1 : nesl_utility/PS-Simulink Converter  PhysicalDomain=network_engine_domain  SubClassName=ps_output  LeftPortType=input  RightPortType=output  PseudoPeriodic=off  Frequencies=[]  Unit=1  AffineConversion=off
  PS-Simulink Converter2 : nesl_utility/PS-Simulink Converter  PhysicalDomain=network_engine_domain  SubClassName=ps_output  LeftPortType=input  RightPortType=output  PseudoPeriodic=off  Frequencies=[]  Unit=1  AffineConversion=off
  PS-Simulink Converter3 : nesl_utility/PS-Simulink Converter  PhysicalDomain=network_engine_domain  SubClassName=ps_output  LeftPortType=input  RightPortType=output  PseudoPeriodic=off  Frequencies=[]  Unit=1  AffineConversion=off
  Product : Product  RndMeth=Zero
  Product1 : Product  RndMeth=Zero
  Scope : Scope  NumInputPorts=3
  Simulink-PS Converter : nesl_utility/Simulink-PS Converter  PhysicalDomain=network_engine_domain  SubClassName=ps_input  LeftPortType=input  RightPortType=output  PseudoPeriodic=off  Frequencies=[]  NoiseDistribution=none  NoiseParameters=[]  Unit=1  AffineConversion=off  FilteringAndDerivatives=zero  SimscapeFilterOrder=1  InputFilterTimeConstant=.001  UdotUserProvided=[]
  Simulink-PS Converter1 : nesl_utility/Simulink-PS Converter  PhysicalDomain=network_engine_domain  SubClassName=ps_input  LeftPortType=input  RightPortType=output  PseudoPeriodic=off  Frequencies=[]  NoiseDistribution=none  NoiseParameters=[]  Unit=1  AffineConversion=off  FilteringAndDerivatives=zero  SimscapeFilterOrder=1  InputFilterTimeConstant=.001  UdotUserProvided=[]
  Sum : Sum  Inputs=|++
  To Workspace : ToWorkspace  VariableName=MPCTorqueSwingKnee  SampleTime=-1
  rad2deg : Gain  Gain=180/pi
  "rad2deg1 " : Gain  Gain=180/pi
  w : PMIOPort  Side=Right
  t : PMIOPort  Port=2  Side=Left
  q : PMIOPort  Port=3  Side=Right
  wires:
  PS-Simulink Converter1/1 -> "rad2deg1 "/1
  PS-Simulink Converter2/1 -> rad2deg/1
  rad2deg/1 -> Knee_D_lookup/1, Knee_S_lookup/1, Product/2
  Knee_S_lookup/1 -> Product/1
  "rad2deg1 "/1 -> Product1/1
  Product1/1 -> Sum/1
  Product/1 -> Sum/2
  Sum/1 -> Gain/1
  Knee_D_lookup/1 -> Product1/2
  Gain5/1 -> Add/7
  1-D Lookup Table5/1 -> Gain5/1
  Gain4/1 -> Add/6
  1-D Lookup Table4/1 -> Gain4/1
  Gain3/1 -> Add/5
  1-D Lookup Table3/1 -> Gain3/1
  Gain2/1 -> Add/4
  1-D Lookup Table2/1 -> Gain2/1
  Gain1/1 -> Add/3
  1-D Lookup Table1/1 -> Gain1/1
  Gain6/1 -> Add/2
  1-D Lookup Table/1 -> Gain6/1
  Fcn/1 -> Gain7/1
  Clock/1 -> 1-D Lookup Table/1, 1-D Lookup Table1/1, 1-D Lookup Table2/1, 1-D Lookup Table3/1, 1-D Lookup Table5/1, 1-D Lookup Table4/1, Fcn/1
  Gain/1 -> Scope/2, Simulink-PS Converter1/1
  PS-Simulink Converter3/1 -> Scope/1
  Add/1 -> Simulink-PS Converter/1, Scope/3, To Workspace/1
  Gain7/1 -> Add/1
  connections:
  Hard_Stop_Knee_L1/LConn1 -- PS-Simulink Converter1/LConn1 -- w/RConn1
  Hard_Stop_Knee_L1/RConn1 -- PS-Simulink Converter3/LConn1 -- PS Add/LConn2
  q/RConn1 -- PS-Simulink Converter2/LConn1
  Simulink-PS Converter1/RConn1 -- PS Add1/LConn2
  PS Add/RConn1 -- PS Add1/LConn1
  PS Add1/RConn1 -- t/RConn1
  Simulink-PS Converter/RConn1 -- PS Add/LConn1
